simulink model "Exercise3_SL_Start"  (R2024a)
settings: Solver=FixedStepDiscrete  StartTime=0.0  StopTime=20  RelTol=1e-3
PreLoadFcn:
  | % NXP_MBDT_S32K3 callback: DO NOT REMOVE
  | % mbd_s32k3.common.nxp.model_callbacks.preLoadFcn();
PostLoadFcn:
  | % NXP_MBDT_S32K3 callback: DO NOT REMOVE
  | % mbd_s32k3.common.nxp.model_callbacks.postLoadFcn();
InitFcn:
  | % NXP_MBDT_S32K3 callback: DO NOT REMOVE
  | % mbd_s32k3.common.nxp.model_callbacks.initFcn();
values from neighbouring files (symbols this model uses):
  RShunt = 0.5    [S32K39_CodeGen.sldd]
settings Model: DataDictionary=Exercise1_Data_Solution.sldd  Creator=nxf64875  LastModifiedBy=jharper
settings OptimizationCC: EnhancedBackFolding=on  PassReuseOutputArgsAs=Individual arguments  ZeroExternalMemoryAtStartup=off  ZeroInternalMemoryAtStartup=off  MaxStackSize=64  OptimizeBlockOrder=speed  DifferentSizesBufferReuse=on  OptimizationCustomize=off  EfficientTunableParamExpr=on
settings DebuggingCC: ParameterTunabilityLossMsg=error
settings HardwareCC: ProdBitPerPointer=32  ProdBitPerSizeT=32  ProdBitPerPtrDiffT=32  ProdLargestAtomicInteger=Long  ProdLargestAtomicFloat=Double  ProdWordSize=32  ProdHWDeviceType=ARM Compatible->ARM Cortex
settings ModelReferenceCC: ModelReferenceNumInstancesAllowed=Single
settings SFSimCC: MATLABDynamicMemAlloc=off
settings RTWCC: Description=Embedded Coder  SystemTargetFile=ert.tlc  HardwareBoard=NXP S32K3xx  TemplateMakefile=ert_default_tmf  Toolchain=S32DS GCC  BuildConfiguration=Faster Runs  GPUComputeCapability=3.5
settings CodeAppCC: ForceParamTrailComments=on  IgnoreCustomStorageClasses=off  OperatorAnnotations=on  SimulinkDataObjDesc=on  SFDataObjDesc=on  InsertBlockDesc=on
settings ERTTargetCC: ExtModeTransport=1  ExtModeMexFile=ext_serial_win32_comm  ERTSrcFileBannerTemplate=mbd_s32k3_ert_code_template.cgt  ERTHdrFileBannerTemplate=mbd_s32k3_ert_code_template.cgt  ERTDataSrcFileTemplate=mbd_s32k3_ert_code_template.cgt  ERTDataHdrFileTemplate=mbd_s32k3_ert_code_template.cgt

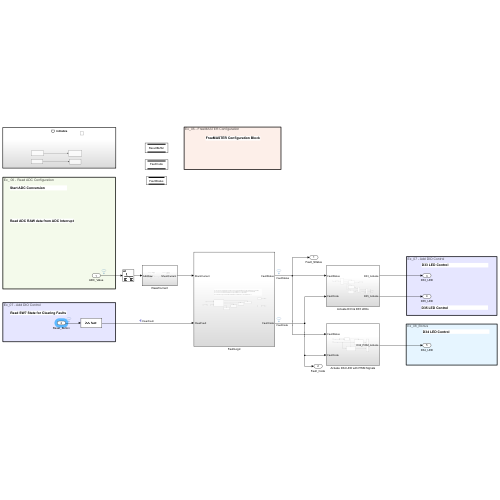
[thumbnail: Simulink's stored preview of the top-level diagram]
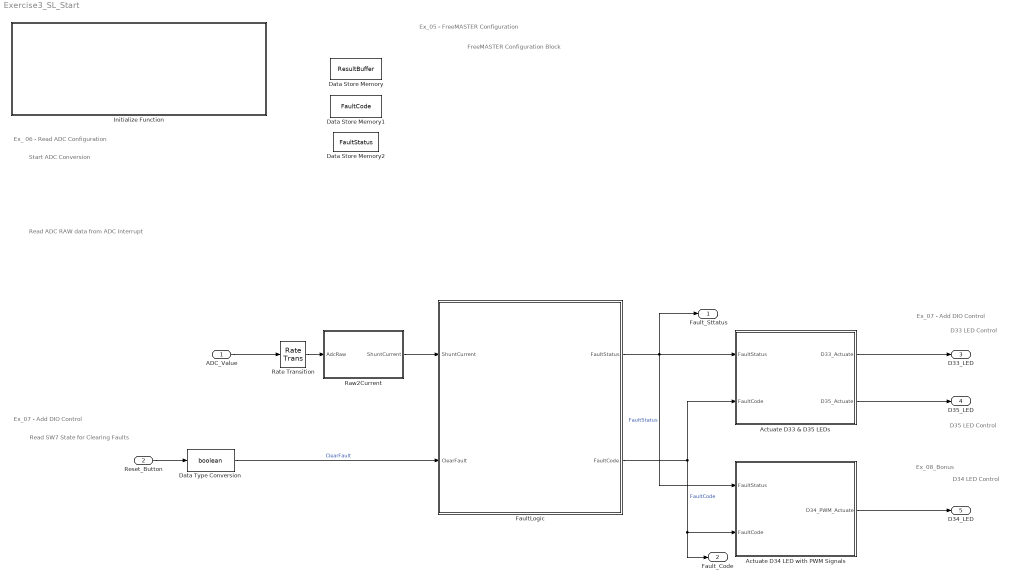
== system Exercise3_SL_Start ==
  note: Ex_05 - FreeMASTER Configuration
  note: Ex_ 06 - Read ADC Configuration
  note: Ex_07 - Add DIO Control
  note: Ex_08_Bonus
  note: FreeMASTER Configuration Block
  note: Start ADC Conversion
  note: Read SW7 State for Clearing Faults
  note: D34 LED Control
  note: Read ADC RAW data from ADC Interrupt
  note: D33 LED Control
  note: D35 LED Control
  note: Ex_07 - Add DIO Control
  ADC_Value : Inport  OutDataTypeStr=single
  Reset_Button : Inport  Port=2  OutDataTypeStr=boolean
  Actuate D33 & D35 LEDs : Subsystem
  Actuate D34 LED with PWM Signals : Subsystem
  Data Store Memory : DataStoreMemory  DataStoreName=ResultBuffer  ReadBeforeWriteMsg=warning  WriteAfterWriteMsg=warning  WriteAfterReadMsg=warning  ShowAdditionalParam=off  OutDataTypeStr=uint16
  Data Store Memory1 : DataStoreMemory  DataStoreName=FaultCode  WriteAfterWriteMsg=warning  InitialValue=int16(0)  ShowAdditionalParam=off  OutMin=0  OutMax=3  OutDataTypeStr=int16
  Data Store Memory2 : DataStoreMemory  DataStoreName=FaultStatus  WriteAfterWriteMsg=warning  InitialValue=false  ShowAdditionalParam=off  OutDataTypeStr=boolean
  Data Type Conversion : DataTypeConversion  OutDataTypeStr=boolean  SaturateOnIntegerOverflow=off  RndMeth=Floor
  FaultLogic : Subsystem
  Initialize Function : Subsystem  TreatAsAtomicUnit=on
  Rate Transition : RateTransition
  Raw2Current : Subsystem
  Fault_Sttatus : Outport
  Fault_Code : Outport  Port=2
  D33_LED : Outport  Port=3
  D35_LED : Outport  Port=4
  D34_LED : Outport  Port=5
  wires:
  Data Type Conversion/1 -> FaultLogic/2(ClearFault)  "ClearFault"
  ADC_Value/1 -> Rate Transition/1
  FaultLogic/1(FaultStatus) -> Fault_Sttatus/1, Actuate D34 LED with PWM Signals/1(FaultStatus), Actuate D33 & D35 LEDs/1(FaultStatus)  "FaultStatus"
  Raw2Current/1(ShuntCurrent) -> FaultLogic/1(ShuntCurrent)
  Rate Transition/1 -> Raw2Current/1(AdcRaw)
  Reset_Button/1 -> Data Type Conversion/1
  FaultLogic/2(FaultCode) -> Fault_Code/1, Actuate D34 LED with PWM Signals/2(FaultCode), Actuate D33 & D35 LEDs/2(FaultCode)  "FaultCode"
  Actuate D34 LED with PWM Signals/1(D34_PWM_Actuate) -> D34_LED/1
  Actuate D33 & D35 LEDs/2(D35_Actuate) -> D35_LED/1
  Actuate D33 & D35 LEDs/1(D33_Actuate) -> D33_LED/1

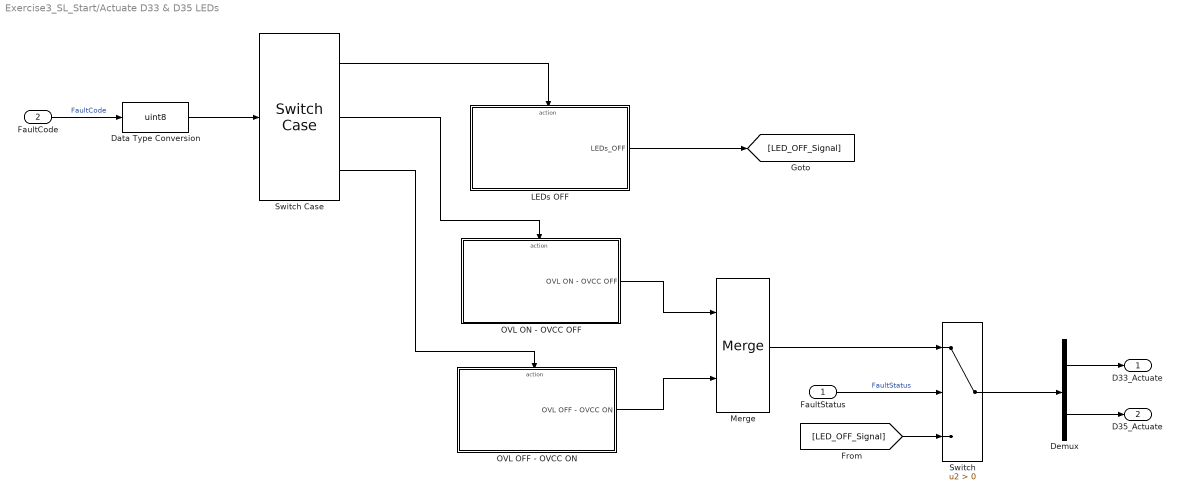
== system Exercise3_SL_Start/Actuate D33 & D35 LEDs ==
  FaultStatus : Inport
  FaultCode : Inport  Port=2
  Data Type Conversion : DataTypeConversion  OutDataTypeStr=uint8  SaturateOnIntegerOverflow=off  RndMeth=Floor
  Demux : Demux  Outputs=2
  LEDs OFF : Subsystem  TreatAsAtomicUnit=on
  Merge : Merge
  OVL OFF - OVCC ON : Subsystem  TreatAsAtomicUnit=on
  OVL ON - OVCC OFF : Subsystem  TreatAsAtomicUnit=on
  Switch : Switch  Criteria=u2 > Threshold  SaturateOnIntegerOverflow=off  InputSameDT=off
  Switch Case : SwitchCase  CaseConditions={0,2,3}  ShowDefaultCase=off
  D33_Actuate : Outport
  D35_Actuate : Outport  Port=2
  wires:
  Switch Case/2 -> OVL ON - OVCC OFF/Action
  Switch Case/1 -> LEDs OFF/Action
  FaultStatus/1 -> Switch/2  "FaultStatus"
  FaultCode/1 -> Data Type Conversion/1  "FaultCode"
  Switch/1 -> Demux/1
  Demux/2 -> D35_Actuate/1
  Demux/1 -> D33_Actuate/1
  Switch Case/3 -> OVL OFF - OVCC ON/Action
  Data Type Conversion/1 -> Switch Case/1
  OVL ON - OVCC OFF/1(OVL ON - OVCC OFF) -> Merge/1
  OVL OFF - OVCC ON/1(OVL OFF - OVCC ON) -> Merge/2
  Merge/1 -> Switch/1
  LEDs OFF/1(LEDs_OFF) -> [LED_OFF_Signal]
  [LED_OFF_Signal] -> Switch/3

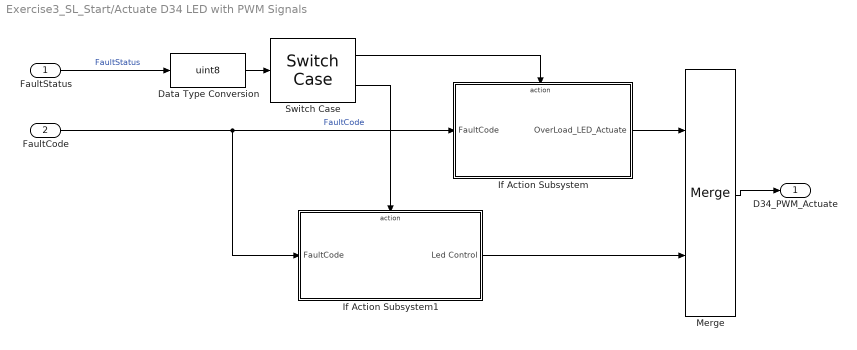
== system Exercise3_SL_Start/Actuate D34 LED with PWM Signals ==
  FaultStatus : Inport
  FaultCode : Inport  Port=2
  Data Type Conversion : DataTypeConversion  OutDataTypeStr=uint8  SaturateOnIntegerOverflow=off  RndMeth=Floor
  If Action Subsystem : Subsystem  TreatAsAtomicUnit=on
  If Action Subsystem1 : Subsystem  TreatAsAtomicUnit=on
  Merge : Merge
  Switch Case : SwitchCase  CaseConditions={0,1}  ShowDefaultCase=off
  D34_PWM_Actuate : Outport
  wires:
  FaultCode/1 -> If Action Subsystem1/1(FaultCode), If Action Subsystem/1(FaultCode)  "FaultCode"
  Switch Case/2 -> If Action Subsystem1/Action
  Merge/1 -> D34_PWM_Actuate/1
  If Action Subsystem/1(OverLoad_LED_Actuate) -> Merge/1
  Data Type Conversion/1 -> Switch Case/1
  Switch Case/1 -> If Action Subsystem/Action
  FaultStatus/1 -> Data Type Conversion/1  "FaultStatus"
  If Action Subsystem1/1(Led Control) -> Merge/2

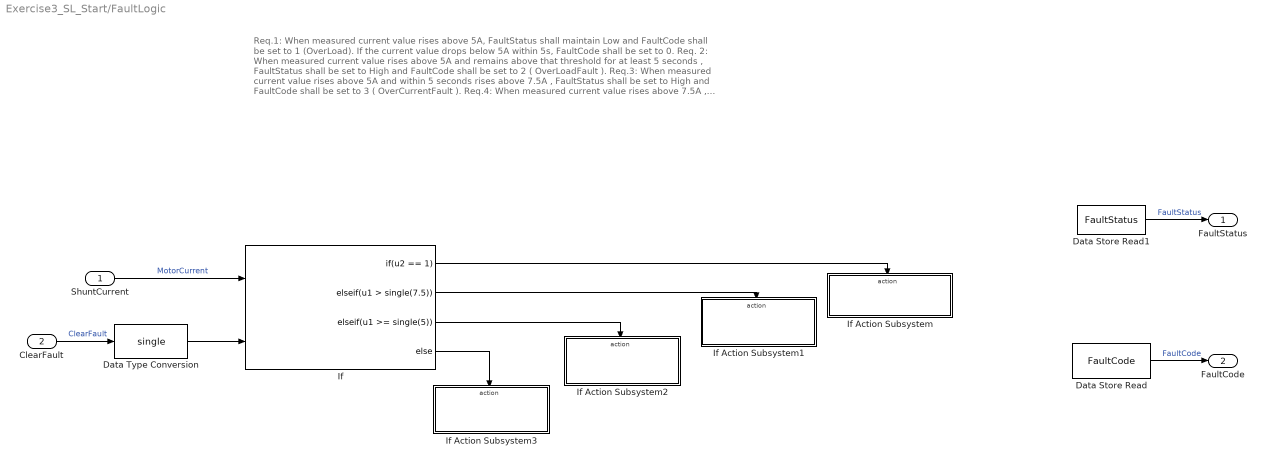
== system Exercise3_SL_Start/FaultLogic ==
  note: Req.1: When measured current value rises above 5A, FaultStatus shall maintain Low and FaultCode shall be set to 1 (OverLoad). If the current value drops below 5A within 5s, FaultCode shall be set to 0.
      |
      | Req. 2: When measured current value rises above 5A and remains above that threshold for at least 5 seconds , FaultStatus shall be set to High and FaultCode shall be set to 2 ( OverLoadFault ).
      |
      | Req.3: When measured current value rises above 5A and within 5 seconds rises above 7.5A , FaultStatus shall be set to High and FaultCode shall be set to 3 ( OverCurrentFault ).
      |
      | Req.4: When measured current value rises above 7.5A , FaultStatus shall be set to High and FaultCode shall be set to 3 ( OverCurrentFault ).
      |
      | Req.5: When ClearFault is set to High while either OverLoadFault or OverCurrentFault is active, FaultStatus shall be set to Low and FaultCode shall be set to 0.
  ShuntCurrent : Inport  OutDataTypeStr=single  Unit=V  PortDimensions=1  SampleTime=0.001
  ClearFault : Inport  Port=2  OutDataTypeStr=boolean  PortDimensions=1  SampleTime=0.001
  Data Store Read : DataStoreRead  Priority=2  DataStoreName=FaultCode  IndexOptions=Index vector (dialog)  Indices=1  OutputSizes=1
  Data Store Read1 : DataStoreRead  Priority=2  DataStoreName=FaultStatus  IndexOptions=Index vector (dialog)  Indices=1  OutputSizes=1
  Data Type Conversion : DataTypeConversion  OutDataTypeStr=single  SaturateOnIntegerOverflow=off  RndMeth=Floor
  If : If  Priority=1  NumInputs=2  IfExpression=u2 == 1  ElseIfExpressions=u1 > single(7.5), u1 >= single(5)
  If Action Subsystem : Subsystem  TreatAsAtomicUnit=on
  If Action Subsystem1 : Subsystem  TreatAsAtomicUnit=on
  If Action Subsystem2 : Subsystem  TreatAsAtomicUnit=on
  If Action Subsystem3 : Subsystem  TreatAsAtomicUnit=on
  FaultStatus : Outport  OutDataTypeStr=boolean
  FaultCode : Outport  Port=2  OutDataTypeStr=int16
  wires:
  Data Store Read1/1 -> FaultStatus/1  "FaultStatus"
  ShuntCurrent/1 -> If/1  "MotorCurrent"
  Data Store Read/1 -> FaultCode/1  "FaultCode"
  ClearFault/1 -> Data Type Conversion/1  "ClearFault"
  If/1 -> If Action Subsystem/Action
  If/2 -> If Action Subsystem1/Action
  Data Type Conversion/1 -> If/2
  If/3 -> If Action Subsystem2/Action
  If/4 -> If Action Subsystem3/Action

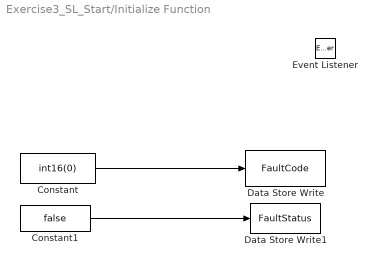
== system Exercise3_SL_Start/Initialize Function ==
  Constant : Constant  Value=int16(0)  OutDataTypeStr=int16
  Constant1 : Constant  Value=false  OutDataTypeStr=boolean
  Data Store Write : DataStoreWrite  DataStoreName=FaultCode  IndexOptions=Index vector (dialog)  Indices=1  OutputSizes=1
  Data Store Write1 : DataStoreWrite  DataStoreName=FaultStatus  IndexOptions=Index vector (dialog)  Indices=1  OutputSizes=1
  Event Listener : EventListener  DisableCoverage=on  EventName=reset
  wires:
  Constant1/1 -> Data Store Write1/1
  Constant/1 -> Data Store Write/1

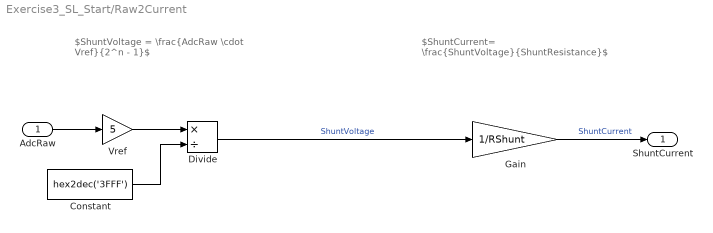
== system Exercise3_SL_Start/Raw2Current ==
  note: $ShuntVoltage = \frac{AdcRaw \cdot Vref}{2^n - 1}$
  note: $ShuntCurrent= \frac{ShuntVoltage}{ShuntResistance}$
  AdcRaw : Inport
  Constant : Constant  Value=hex2dec('3FFF')  OutDataTypeStr=single
  Divide : Product  Inputs=*/  OutDataTypeStr=single
  Gain : Gain  Gain=1/RShunt  OutDataTypeStr=single
  Vref : Gain  Gain=5
  ShuntCurrent : Outport
  wires:
  Vref/1 -> Divide/1
  Constant/1 -> Divide/2
  AdcRaw/1 -> Vref/1
  Divide/1 -> Gain/1  "ShuntVoltage"
  Gain/1 -> ShuntCurrent/1  "ShuntCurrent"

== system Exercise3_SL_Start/Actuate D33 & D35 LEDs/LEDs OFF ==
  Action Port : ActionPort  ActionPortLabel=case [ 0 ]:
  Constant1 : Constant  Value=0  OutDataTypeStr=uint8
  Constant2 : Constant  Value=0  OutDataTypeStr=uint8
  Mux : Mux  Inputs=2
  LEDs_OFF : Outport  InitialOutput=[0 0]
  wires:
  Mux/1 -> LEDs_OFF/1
  Constant1/1 -> Mux/1
  Constant2/1 -> Mux/2

== system Exercise3_SL_Start/Actuate D33 & D35 LEDs/OVL OFF - OVCC ON ==
  Action Port : ActionPort  ActionPortLabel=case [ 3 ]:
  Constant1 : Constant  Value=0  OutDataTypeStr=uint8
  Constant2 : Constant  OutDataTypeStr=uint8
  Mux : Mux  Inputs=2
  OVL OFF - OVCC ON : Outport  InitialOutput=[0 1]
  wires:
  Mux/1 -> OVL OFF - OVCC ON/1
  Constant1/1 -> Mux/1
  Constant2/1 -> Mux/2

== system Exercise3_SL_Start/Actuate D33 & D35 LEDs/OVL ON - OVCC OFF ==
  Action Port : ActionPort  ActionPortLabel=case [ 2 ]:
  Constant1 : Constant  OutDataTypeStr=uint8
  Constant2 : Constant  Value=0  OutDataTypeStr=uint8
  Mux : Mux  Inputs=2
  OVL ON - OVCC OFF : Outport  InitialOutput=[1 0]
  wires:
  Mux/1 -> OVL ON - OVCC OFF/1
  Constant1/1 -> Mux/1
  Constant2/1 -> Mux/2

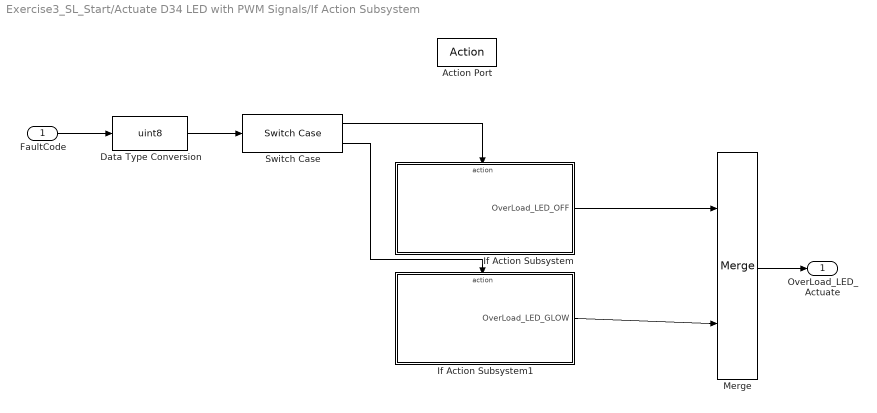
== system Exercise3_SL_Start/Actuate D34 LED with PWM Signals/If Action Subsystem ==
  FaultCode : Inport
  Action Port : ActionPort  ActionPortLabel=case [ 0 ]:
  Data Type Conversion : DataTypeConversion  OutDataTypeStr=uint8  SaturateOnIntegerOverflow=off  RndMeth=Floor
  If Action Subsystem : Subsystem  TreatAsAtomicUnit=on
  If Action Subsystem1 : Subsystem  TreatAsAtomicUnit=on
  Merge : Merge
  Switch Case : SwitchCase  CaseConditions={0,1}  ShowDefaultCase=off
  OverLoad_LED_Actuate : Outport
  wires:
  Switch Case/2 -> If Action Subsystem1/Action
  Switch Case/1 -> If Action Subsystem/Action
  Data Type Conversion/1 -> Switch Case/1
  FaultCode/1 -> Data Type Conversion/1
  If Action Subsystem/1(OverLoad_LED_OFF) -> Merge/1
  Merge/1 -> OverLoad_LED_Actuate/1
  If Action Subsystem1/1(OverLoad_LED_GLOW) -> Merge/2

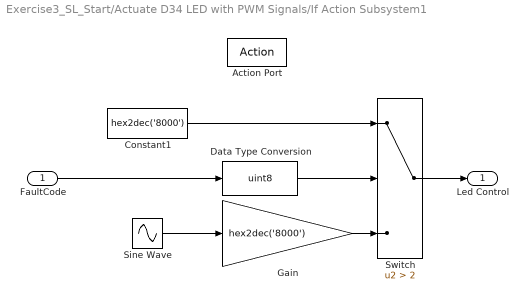
== system Exercise3_SL_Start/Actuate D34 LED with PWM Signals/If Action Subsystem1 ==
  FaultCode : Inport
  Action Port : ActionPort  ActionPortLabel=case [ 1 ]:
  Constant1 : Constant  Value=hex2dec('8000')  OutDataTypeStr=uint16
  Data Type Conversion : DataTypeConversion  OutDataTypeStr=uint8  SaturateOnIntegerOverflow=off  RndMeth=Floor
  Gain : Gain  Gain=hex2dec('8000')  OutDataTypeStr=uint16
  Sine Wave : Sin  Amplitude=0.5  Bias=0.5  Frequency=4*pi
  Switch : Switch  Criteria=u2 > Threshold  Threshold=2  SaturateOnIntegerOverflow=off  InputSameDT=off
  Led Control : Outport
  wires:
  FaultCode/1 -> Data Type Conversion/1
  Gain/1 -> Switch/3
  Sine Wave/1 -> Gain/1
  Constant1/1 -> Switch/1
  Switch/1 -> Led Control/1
  Data Type Conversion/1 -> Switch/2

== system Exercise3_SL_Start/FaultLogic/If Action Subsystem ==
  Action Port : ActionPort  ActionPortLabel=if(u2 == 1)
  Constant : Constant  Value=int16(0)  OutDataTypeStr=int16
  Constant1 : Constant  Value=false  OutDataTypeStr=boolean
  Data Store Write : DataStoreWrite  DataStoreName=FaultCode  IndexOptions=Index vector (dialog)  Indices=1  OutputSizes=1
  Data Store Write1 : DataStoreWrite  DataStoreName=FaultStatus  IndexOptions=Index vector (dialog)  Indices=1  OutputSizes=1
  wires:
  Constant/1 -> Data Store Write/1
  Constant1/1 -> Data Store Write1/1

== system Exercise3_SL_Start/FaultLogic/If Action Subsystem1 ==
  Action Port : ActionPort  ActionPortLabel=elseif(u1 > single(7.5))
  Constant : Constant  Value=int16(3)  OutDataTypeStr=int16
  Constant1 : Constant  Value=true  OutDataTypeStr=boolean
  Data Store Write : DataStoreWrite  DataStoreName=FaultCode  IndexOptions=Index vector (dialog)  Indices=1  OutputSizes=1
  Data Store Write1 : DataStoreWrite  DataStoreName=FaultStatus  IndexOptions=Index vector (dialog)  Indices=1  OutputSizes=1
  wires:
  Constant1/1 -> Data Store Write1/1
  Constant/1 -> Data Store Write/1

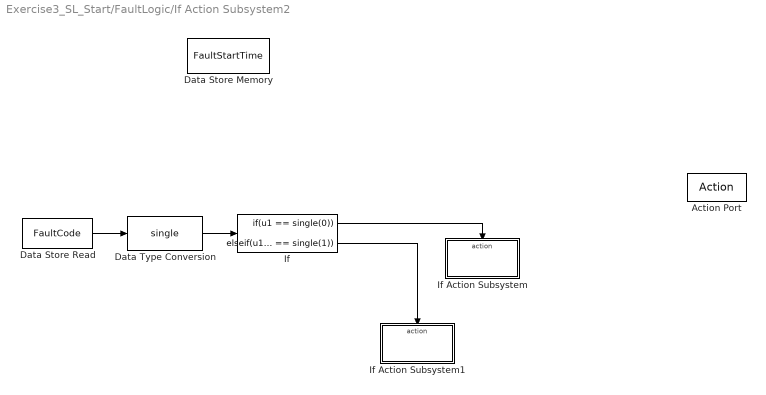
== system Exercise3_SL_Start/FaultLogic/If Action Subsystem2 ==
  Action Port : ActionPort  ActionPortLabel=elseif( u1 >= single(5))
  Data Store Memory : DataStoreMemory  DataStoreName=FaultStartTime  WriteAfterWriteMsg=warning  ShowAdditionalParam=off  OutDataTypeStr=double
  Data Store Read : DataStoreRead  DataStoreName=FaultCode  IndexOptions=Index vector (dialog)  Indices=1  OutputSizes=1
  Data Type Conversion : DataTypeConversion  OutDataTypeStr=single  SaturateOnIntegerOverflow=off  RndMeth=Floor
  If : If  IfExpression=u1 == single(0)  ElseIfExpressions=u1 == single(1)  ShowElse=off
  If Action Subsystem : Subsystem  TreatAsAtomicUnit=on
  If Action Subsystem1 : Subsystem  TreatAsAtomicUnit=on
  wires:
  If/1 -> If Action Subsystem/Action
  Data Type Conversion/1 -> If/1
  Data Store Read/1 -> Data Type Conversion/1
  If/2 -> If Action Subsystem1/Action

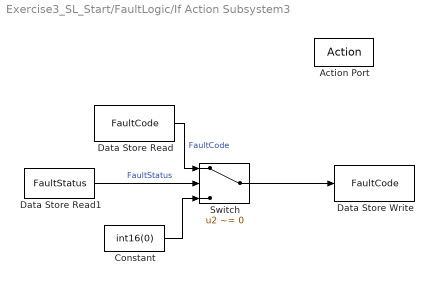
== system Exercise3_SL_Start/FaultLogic/If Action Subsystem3 ==
  Action Port : ActionPort  ActionPortLabel=else
  Constant : Constant  Value=int16(0)
  Data Store Read : DataStoreRead  Priority=2  DataStoreName=FaultCode  IndexOptions=Index vector (dialog)  Indices=1  OutputSizes=1
  Data Store Read1 : DataStoreRead  Priority=2  DataStoreName=FaultStatus  IndexOptions=Index vector (dialog)  Indices=1  OutputSizes=1
  Data Store Write : DataStoreWrite  DataStoreName=FaultCode  IndexOptions=Index vector (dialog)  Indices=1  OutputSizes=1
  Switch : Switch  Criteria=u2 ~= 0  SaturateOnIntegerOverflow=off  InputSameDT=off
  wires:
  Data Store Read1/1 -> Switch/2  "FaultStatus"
  Data Store Read/1 -> Switch/1  "FaultCode"
  Switch/1 -> Data Store Write/1
  Constant/1 -> Switch/3

== system Exercise3_SL_Start/Actuate D34 LED with PWM Signals/If Action Subsystem/If Action Subsystem ==
  Action Port : ActionPort  ActionPortLabel=case [ 0 ]:
  Constant1 : Constant  Value=0  OutDataTypeStr=uint16
  OverLoad_LED_OFF : Outport
  wires:
  Constant1/1 -> OverLoad_LED_OFF/1

== system Exercise3_SL_Start/Actuate D34 LED with PWM Signals/If Action Subsystem/If Action Subsystem1 ==
  Action Port : ActionPort  ActionPortLabel=case [ 1 ]:
  Gain : Gain  Gain=hex2dec('8000')  OutDataTypeStr=uint16
  Sine Wave : Sin  Amplitude=0.5  Bias=0.5  Frequency=pi
  OverLoad_LED_GLOW : Outport
  wires:
  Gain/1 -> OverLoad_LED_GLOW/1
  Sine Wave/1 -> Gain/1

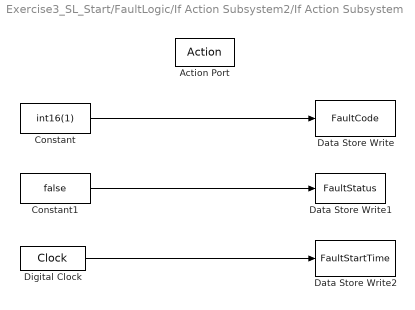
== system Exercise3_SL_Start/FaultLogic/If Action Subsystem2/If Action Subsystem ==
  Action Port : ActionPort  ActionPortLabel=if(u1 == single(0))
  Constant : Constant  Value=int16(1)  OutDataTypeStr=int16
  Constant1 : Constant  Value=false  OutDataTypeStr=boolean
  Data Store Write : DataStoreWrite  DataStoreName=FaultCode  IndexOptions=Index vector (dialog)  Indices=1  OutputSizes=1
  Data Store Write1 : DataStoreWrite  DataStoreName=FaultStatus  IndexOptions=Index vector (dialog)  Indices=1  OutputSizes=1
  Data Store Write2 : DataStoreWrite  DataStoreName=FaultStartTime  IndexOptions=Index vector (dialog)  Indices=1  OutputSizes=1
  Digital Clock : DigitalClock  SampleTime=0.001
  wires:
  Constant1/1 -> Data Store Write1/1
  Constant/1 -> Data Store Write/1
  Digital Clock/1 -> Data Store Write2/1

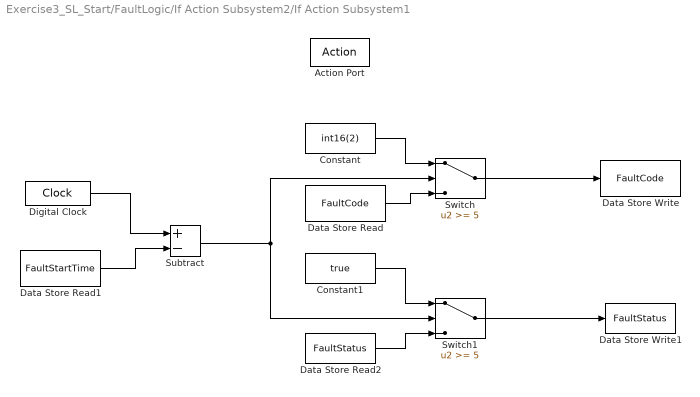
== system Exercise3_SL_Start/FaultLogic/If Action Subsystem2/If Action Subsystem1 ==
  Action Port : ActionPort  ActionPortLabel=elseif(u1 == single(1))
  Constant : Constant  Value=int16(2)  OutDataTypeStr=int16
  Constant1 : Constant  Value=true  OutDataTypeStr=boolean
  Data Store Read : DataStoreRead  DataStoreName=FaultCode  IndexOptions=Index vector (dialog)  Indices=1  OutputSizes=1
  Data Store Read1 : DataStoreRead  DataStoreName=FaultStartTime  IndexOptions=Index vector (dialog)  Indices=1  OutputSizes=1
  Data Store Read2 : DataStoreRead  DataStoreName=FaultStatus  IndexOptions=Index vector (dialog)  Indices=1  OutputSizes=1
  Data Store Write : DataStoreWrite  DataStoreName=FaultCode  IndexOptions=Index vector (dialog)  Indices=1  OutputSizes=1
  Data Store Write1 : DataStoreWrite  DataStoreName=FaultStatus  IndexOptions=Index vector (dialog)  Indices=1  OutputSizes=1
  Digital Clock : DigitalClock  SampleTime=0.001
  Subtract : Sum  Inputs=+-
  Switch : Switch  Threshold=5  SaturateOnIntegerOverflow=off  InputSameDT=off
  Switch1 : Switch  Threshold=5  SaturateOnIntegerOverflow=off  InputSameDT=off
  wires:
  Digital Clock/1 -> Subtract/1
  Data Store Read1/1 -> Subtract/2
  Subtract/1 -> Switch1/2, Switch/2
  Constant/1 -> Switch/1
  Constant1/1 -> Switch1/1
  Switch/1 -> Data Store Write/1
  Switch1/1 -> Data Store Write1/1
  Data Store Read/1 -> Switch/3
  Data Store Read2/1 -> Switch1/3
